simulink model "realistic_closed_loop_system"  (R2025b)
settings: Solver=ode5  StartTime=0.0  StopTime=10.0  RelTol=1e-3
values from neighbouring files (symbols this model uses):
  A = [0 0 0 0 0 0 -4.52769230769 47.0088272383 1 0 -16.8834805098 55.3556738027 ... (16 elements, 4x4)]    [angle_sensor_data.mat]    (also in freq_experiments.m = [0, 0, 1, 0; inv_pend.m = [0, 0, 1, 0; lqr_tuning.m = [0, 0, 1, 0; position_sensor_data.mat)
  B = [0 0 3.77779700614 -12.3862196923]    [angle_sensor_data.mat]    (also in freq_experiments.m = [0; 0; (Km*Kg)/(M*Rm*r); (-Km*Kg)/(r*Rm*M*l)]; inv_pend.m = [0; 0; (Km*Kg)/(M*Rm*r); (-Km*Kg)/(r*Rm*M*l)]; lqr_tuning.m = [0; 0; (Km*Kg)/(M*Rm*r); (-Km*Kg)/(r*Rm*M*l)]; position_sensor_data.mat)
  Fa = 0.248229508027    [angle_sensor_data.mat]    (also in freq_experiments.m; inv_pend.m; lqr_tuning.m; position_sensor_data.mat)
  Fx = 0.103401360544    [angle_sensor_data.mat]    (also in freq_experiments.m; inv_pend.m; lqr_tuning.m; position_sensor_data.mat)
  K = [-18.2574185835 -93.1723220187 -24.9464299712 -21.1521187188]    [angle_sensor_data.mat]    (also in freq_experiments.m = lqr(A, B, Q, R); inv_pend.m = lqr(A, B, Q, R); lqr_tuning.m = lqr(A,B,Q,R); position_sensor_data.mat)
  Ts = 0.005    [angle_sensor_data.mat]    (also in freq_experiments.m; inv_pend.m; lqr_tuning.m; position_sensor_data.mat)
  Wc = 31.4159265359    [angle_sensor_data.mat]    (also in freq_experiments.m; inv_pend.m; lqr_tuning.m; position_sensor_data.mat)
settings Model: Creator=sm  LastModifiedBy=sm
settings HardwareCC: ProdBitPerLong=64.0  ProdHWDeviceType=Intel->x86-64 (Linux 64)
settings RTWCC: SystemTargetFile=sldrt.tlc  TemplateMakefile=sldrt.tmf  RTWCompilerOptimization=on  Description=Simulink Desktop Real-Time
settings CodeAppCC: MaxIdLength=95.0
settings SimulinkDesktopRealTimeCC: ExtModeTransport=0.0  ExtModeStaticAllocSize=1000000.0  TargetLibSuffix=_sldrt.a  TargetPreCompLibLocation=/usr/local/MATLAB/R2025b/toolbox/sldrt/lib/glnxa64  MultiwordLength=2048.0  DynamicStringBufferSize=256.0  ParMdlRefBuildCompliant=on  PreserveMATLABNamespacesInGeneratedCode=on  SubcomponentCodeInterfacePackaging=Reusable function

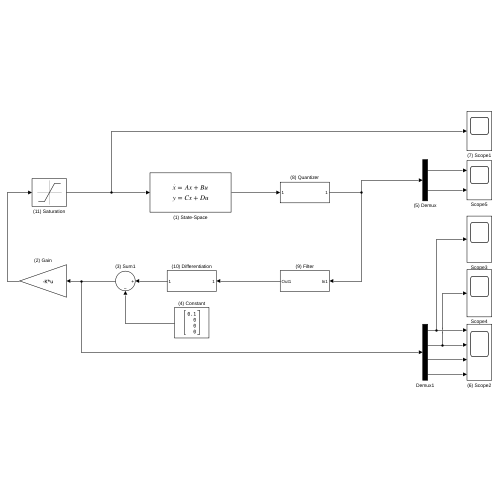
[thumbnail: Simulink's stored preview of the top-level diagram]
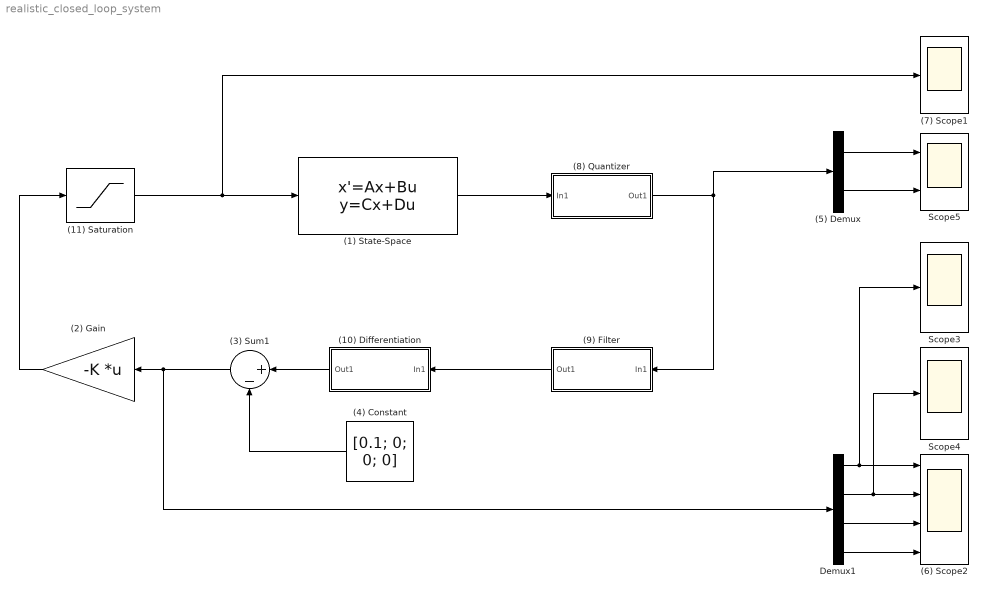
== system realistic_closed_loop_system ==
  (1) State-Space : StateSpace  A=A  B=B  C=[1, 0, 0, 0; 0, 1, 0, 0]  D=zeros(2,1)  InitialCondition=[0; 0; 0; 0]
  (10) Differentiation : Subsystem
  (11) Saturation : Saturate  UpperLimit=5  LowerLimit=-5
  (2) Gain : Gain  Gain=-K  Multiplication=Matrix(K*u)
  (3) Sum1 : Sum  Inputs=|+-
  (4) Constant : Constant  Value=[0.1; 0; 0; 0]  VectorParams1D=off
  (5) Demux : Demux  Outputs=2
  (6) Scope2 : Scope  NumInputPorts=4
      settings: Title=Filtered Anglular Position [rad]  ActiveDisplayYMinimum=-0.64808142081073672  ActiveDisplayYMaximum=0.37740044873205181  DataLoggingVariableName=realistic
  (7) Scope1 : Scope
      settings: Title=Voltage [V]  ActiveDisplayYMinimum=-24.163791154276673  ActiveDisplayYMaximum=34.351697914703692  DataLoggingVariableName=step_voltage
  (8) Quantizer : Subsystem
  (9) Filter : Subsystem
  Demux1 : Demux
  Scope3 : Scope
      settings: Title=Position [m]  ActiveDisplayYMinimum=-0.49638590354123546  ActiveDisplayYMaximum=0.37029122035074558  DataLoggingVariableName=position_sys_cl
  Scope4 : Scope
      settings: Title=Angular Position [rad]  ActiveDisplayYMinimum=-0.44934447769521407  ActiveDisplayYMaximum=0.27301308046784717  DataLoggingVariableName=angle_step
  Scope5 : Scope  NumInputPorts=2
      settings: Title=Angular position [rad]  ActiveDisplayYMinimum=-24.163791154276673  ActiveDisplayYMaximum=34.351697914703692  DataLoggingVariableName=step_voltage1
  wires:
  Demux1/1 -> Scope3/1, (6) Scope2/1
  Demux1/2 -> Scope4/1, (6) Scope2/2
  Demux1/3 -> (6) Scope2/3
  Demux1/4 -> (6) Scope2/4
  (11) Saturation/1 -> (7) Scope1/1, (1) State-Space/1
  (9) Filter/1(Out1) -> (10) Differentiation/1(In1)
  (8) Quantizer/1(Out1) -> (5) Demux/1, (9) Filter/1(In1)
  (1) State-Space/1 -> (8) Quantizer/1(In1)
  (5) Demux/1 -> Scope5/1
  (5) Demux/2 -> Scope5/2
  (2) Gain/1 -> (11) Saturation/1
  (10) Differentiation/1(Out1) -> (3) Sum1/1
  (3) Sum1/1 -> Demux1/1, (2) Gain/1
  (4) Constant/1 -> (3) Sum1/2

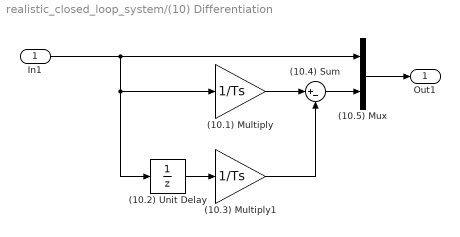
== system realistic_closed_loop_system/(10) Differentiation ==
  In1 : Inport
  (10.1) Multiply : Gain  Gain=1/Ts
  (10.2) Unit Delay : UnitDelay  InitialCondition=[0; 0]  SampleTime=0.005  HasFrameUpgradeWarning=on
  (10.3) Multiply1 : Gain  Gain=1/Ts
  (10.4) Sum : Sum  Inputs=|+-
  (10.5) Mux : Mux  Inputs=2
  Out1 : Outport
  wires:
  (10.5) Mux/1 -> Out1/1
  (10.3) Multiply1/1 -> (10.4) Sum/2
  (10.1) Multiply/1 -> (10.4) Sum/1
  (10.4) Sum/1 -> (10.5) Mux/2
  (10.2) Unit Delay/1 -> (10.3) Multiply1/1
  In1/1 -> (10.2) Unit Delay/1, (10.1) Multiply/1, (10.5) Mux/1

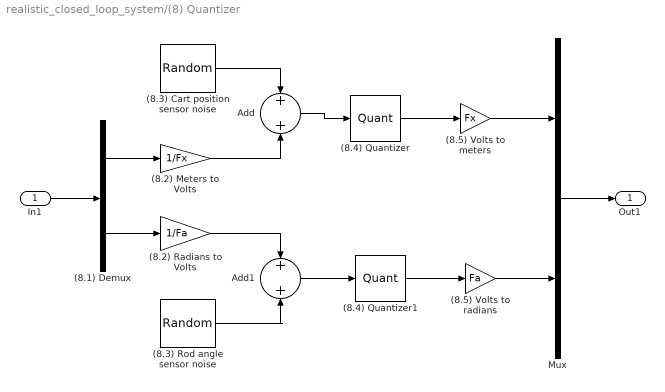
== system realistic_closed_loop_system/(8) Quantizer ==
  In1 : Inport
  " Mux" : Mux  Inputs=2
  (8.1) Demux : Demux  Outputs=2
  (8.2) Meters to Volts : Gain  Gain=1/Fx
  (8.2) Radians to Volts : Gain  Gain=1/Fa
  (8.3) Cart position sensor noise : RandomNumber  Variance=10^-9  Seed=1  SampleTime=0.005
  "(8.3) Rod angle sensor noise " : RandomNumber  Variance=10^-9  Seed=2  SampleTime=0.005
  (8.4) Quantizer : Quantizer  QuantizationInterval=20/2^16
  (8.4) Quantizer1 : Quantizer  QuantizationInterval=20/2^16
  (8.5) Volts to meters : Gain  Gain=Fx
  (8.5) Volts to radians : Gain  Gain=Fa
  Add : Sum
  Add1 : Sum
  Out1 : Outport
  wires:
  " Mux"/1 -> Out1/1
  In1/1 -> (8.1) Demux/1
  (8.1) Demux/1 -> (8.2) Meters to Volts/1
  (8.1) Demux/2 -> (8.2) Radians to Volts/1
  (8.3) Cart position sensor noise/1 -> Add/1
  (8.2) Meters to Volts/1 -> Add/2
  (8.2) Radians to Volts/1 -> Add1/1
  "(8.3) Rod angle sensor noise "/1 -> Add1/2
  Add/1 -> (8.4) Quantizer/1
  (8.4) Quantizer/1 -> (8.5) Volts to meters/1
  (8.5) Volts to meters/1 -> " Mux"/1
  Add1/1 -> (8.4) Quantizer1/1
  (8.4) Quantizer1/1 -> (8.5) Volts to radians/1
  (8.5) Volts to radians/1 -> " Mux"/2

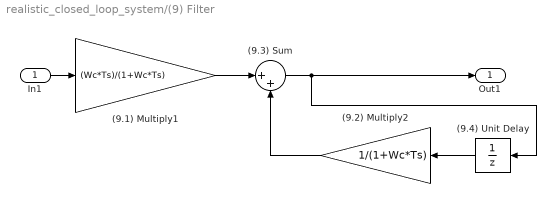
== system realistic_closed_loop_system/(9) Filter ==
  In1 : Inport
  (9.1) Multiply1 : Gain  Gain=(Wc*Ts)/(1+Wc*Ts)
  (9.2) Multiply2 : Gain  Gain=1/(1+Wc*Ts)
  (9.3) Sum : Sum  Inputs=|++
  (9.4) Unit Delay : UnitDelay  InitialCondition=[0; 0]  SampleTime=0.005  HasFrameUpgradeWarning=on
  Out1 : Outport
  wires:
  (9.4) Unit Delay/1 -> (9.2) Multiply2/1
  (9.2) Multiply2/1 -> (9.3) Sum/2
  (9.1) Multiply1/1 -> (9.3) Sum/1
  (9.3) Sum/1 -> Out1/1, (9.4) Unit Delay/1
  In1/1 -> (9.1) Multiply1/1
